simulink model "f2"  (R2021b)
settings: Solver=FixedStepAuto  StartTime=0.0  StopTime=10.0  RelTol=1e-3
libraries: simulink x4
settings Model: Creator=asus  LastModifiedBy=asus

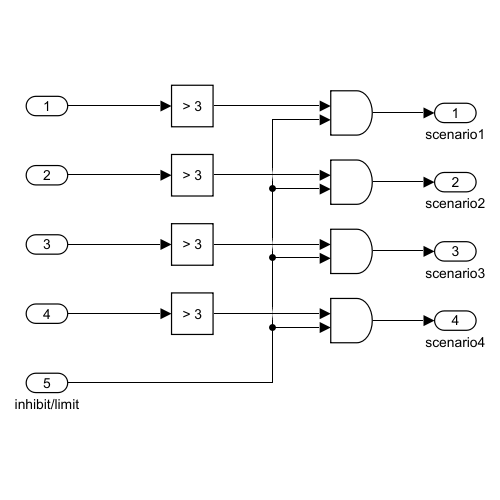
[thumbnail: Simulink's stored preview of the top-level diagram]
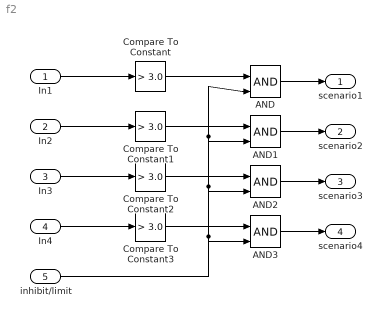
== system f2 ==
  In1 : Inport
  In2 : Inport  Port=2
  In3 : Inport  Port=3
  In4 : Inport  Port=4
  inhibit/limit : Inport  Port=5
  AND{,1..3} (4 alike) : Logic  IconShape=distinctive  AllPortsSameDT=off  OutDataTypeStr=boolean
  Compare To Constant{,1..3} (4 alike) : simulink/Logic and Bit Operations/Compare To Constant  relop=>  const=3.0  OutDataTypeStr=boolean
  scenario1 : Outport
  scenario2 : Outport  Port=2
  scenario3 : Outport  Port=3
  scenario4 : Outport  Port=4
  wires:
  In1/1 -> Compare To Constant/1
  In2/1 -> Compare To Constant1/1
  In4/1 -> Compare To Constant3/1
  In3/1 -> Compare To Constant2/1
  Compare To Constant/1 -> AND/1
  AND/1 -> scenario1/1
  Compare To Constant2/1 -> AND2/1
  Compare To Constant1/1 -> AND1/1
  Compare To Constant3/1 -> AND3/1
  AND1/1 -> scenario2/1
  AND2/1 -> scenario3/1
  AND3/1 -> scenario4/1
  inhibit/limit/1 -> AND3/2, AND2/2, AND1/2, AND/2
